simulink model "engine_rpm_start"  (R2018b)
settings: Solver=ode45  StartTime=0.0  StopTime=50.0  FixedStep=0.001  RelTol=1e-3
PreLoadFcn:
  | load engine_rpm_start.mat
  | Iei = 0.022;
values from neighbouring files (symbols this model uses):
  ENGINE_SPEED = [800 1200 1600 2000 2400 2800 3200 3600 4000 4400 4800]    [engine_rpm.mat]    (also in engine_rpm_start.mat; ex3.mat)
  ENGINE_TORQUE = [-40 215 245 264 264 267 267 267 267 267 -44 117 ... (110 elements, 10x11)]    [engine_rpm.mat]    (also in engine_rpm_start.mat; ex3.mat)
  THROTTLE = [0 20 30 40 50 60 70 80 90 100]    [engine_rpm.mat]    (also in engine_rpm_start.mat; ex3.mat)
undefined symbols (not defined in the file or in its folder): sigbuilder_block
settings Model: Creator=nicholas  LastModifiedBy=yasmine
settings DataIOCC: LimitDataPoints=on  SaveFormat=Array  SignalLoggingName=sigsOut
settings OptimizationCC: BlockReduction=off  BooleanDataType=off  OptimizeBlockIOStorage=off  BufferReuse=off  GlobalBufferReuse=off  ExpressionFolding=off  ExpressionDepthLimit=2147483647  LocalBlockOutputs=off  InitFltsAndDblsToZero=on  LifeSpan=inf  OptimizeDataStoreBuffers=off  BusAssignmentInplaceUpdate=off
settings DebuggingCC: SaveWithParameterizedLinksMsg=none  UnderspecifiedInitializationDetection=Classic  MergeDetectMultiDrivingBlocksExec=none  CheckExecutionContextPreStartOutputMsg=on  CheckExecutionContextRuntimeOutputMsg=on  SignalResolutionControl=TryResolveAllWithWarning  MultiTaskDSMMsg=warning  MultiTaskCondExecSysMsg=none  ParameterPrecisionLossMsg=none  FcnCallInpInsideContextMsg=warning  AllowSymbolicDim=off  StateNameClashWarn=warning  LibraryContextMissingDiagnostic=none  SFUnexpectedBacktrackingDiag=warning  SFNoUnconditionalDefaultTransitionDiag=warning  SFExecutionAtInitializationDiag=none
settings HardwareCC: ProdBitPerPointer=32  ProdBitPerSizeT=32  ProdBitPerPtrDiffT=32  ProdLargestAtomicFloat=None  ProdIntDivRoundTo=Undefined  ProdEndianess=Unspecified  ProdWordSize=32  ProdHWDeviceType=32-bit Generic  TargetUnknown=on
settings ModelReferenceCC: PropagateSignalLabelsOutOfModel=off
settings SFSimCC: SimUseLocalCustomCode=off
settings RTWCC: RTWUseLocalCustomCode=off
settings CodeAppCC: StateflowObjectComments=on
settings GRTTargetCC: TargetFcnLib=ansi_tfl_tmw.mat  TargetLangStandard=C89/C90 (ANSI)  GeneratePreprocessorConditionals=Disable all  CombineOutputUpdateFcns=off  GRTInterface=on
settings ConfigComp: CovMetricSettings=dw  CovHtmlReporting=on  CovSaveCumulativeToWorkspaceVar=on  CovSaveSingleToWorkspaceVar=on  CovExternalEMLEnable=off  CovSFcnEnable=off

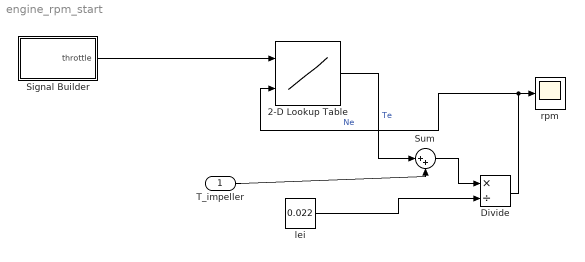
== system engine_rpm_start ==
  T_impeller : Inport
  2-D Lookup Table : Lookup_n-D  BreakpointsForDimension1=THROTTLE  BreakpointsForDimension2=ENGINE_SPEED  Table=ENGINE_TORQUE  InternalRulePriority=Speed  RndMeth=Simplest  InputSameDT=on
  Divide : Product  Inputs=*/
  Signal Builder : Subsystem  Tag=STV Subsys  LoadFcn=sigbuilder_block('load');  StartFcn=sigbuilder_block('start');  StopFcn=sigbuilder_block('stop');  ClipboardFcn=sigbuilder_block('clipboard');  mask(Sigbuilder block){tuvar=[0:10]}
      mask help: Sigbuilder GUI
      mask init:
      | if ~strcmp(get_param(bdroot(gcb),'SimulationStatus'),'stopped') tuvar = sigbuilder_block('maskInit'); end
      settings: CopyFcn=sigbuilder_block('copy');  DeleteFcn=sigbuilder_block('delete');  ModelCloseFcn=sigbuilder_block('modelClose');  PreSaveFcn=sigbuilder_block('preSave');  PauseFcn=sigbuilder_block('pause')  ContinueFcn=sigbuilder_block('continue')  NameChangeFcn=sigbuilder_block('namechange');  OpenFcn=sigbuilder_block('open',[50 50 520 400 ]);  CloseFcn=sigbuilder_block('close');
      mask Display: plot(0, 0, 100, 100,[2, 2, 32, 32, 2], [68, 8, 8, 68, 68],[32, 2], [38, 38], [32, 19, 2],[53, 60, 44], [32, 17, 17, 2],[16, 16, 31, 31]);txt = getActiveGroup(gcbh);text(2, 100, txt,'verticalAlignment', 'top');
  Sum : Sum  Inputs=|++
  lei : Constant  Value=0.022
  rpm : Scope
  wires:
  Signal Builder/1(throttle) -> 2-D Lookup Table/1
  Sum/1 -> Divide/1
  lei/1 -> Divide/2
  Divide/1 -> 2-D Lookup Table/2, rpm/1  "Ne"
  2-D Lookup Table/1 -> Sum/1  "Te"
  T_impeller/1 -> Sum/2

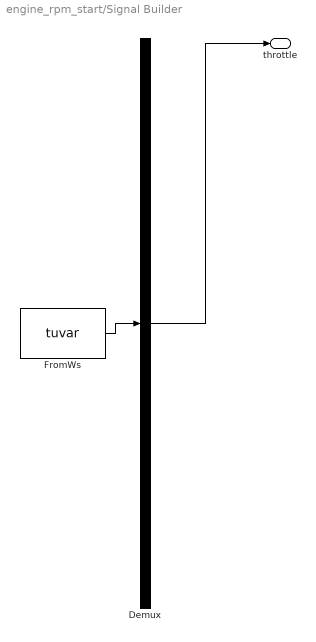
== system engine_rpm_start/Signal Builder ==
  Demux : Demux  Tag=STV Demux  Outputs=1
  FromWs : FromWorkspace  Tag=STV FromWs  VariableName=tuvar  SampleTime=0
      SigBuilderData=|
      | dataSet.timeRange = [0 50]
      | dataSet.name = 'Group 1'
      | sbobj.Groups.Name = 'Group 1'
      | sbobj.Groups.Signals.Name = 'throttle'
      | sbobj.Groups.Signals.XData = [0 15 15 50]
      | sbobj.Groups.Signals.YData = [60 40 100 60]
      | sbobj.Groups.TimeRange = [0 50]
  throttle : Outport  Tag=STV Outport
  wires:
  Demux/1 -> throttle/1
  FromWs/1 -> Demux/1
